simulink model "nieliniowy"  (R2013a)
settings: Solver=ode45  SolverMode=SingleTasking  StartTime=0.0  StopTime=4  RelTol=1e-3
values from neighbouring files (symbols this model uses):
  a = a-b    (= 0.0214)    [model_nielin_zmienne.m]    (also in model_nieliniowy_zmienne.m = 0.0928)
  b = a-b    (= 0.0928)    [model_nielin_zmienne.m]    (also in model_nieliniowy_zmienne.m = 0.0214)
  g = 9.81    [model_nielin_zmienne.m]    (also in model_nieliniowy_zmienne.m)
  k = 0.2607    [model_nielin_zmienne.m]    (also in model_nieliniowy_zmienne.m)
  m = 58    [model_nielin_zmienne.m]    (also in model_nieliniowy_zmienne.m)
  T = 0.024    [model_nielin_zmienne.m]    (also in model_nieliniowy_zmienne.m)
  u_c = -0.0062    [model_nielin_zmienne.m]    (also in model_nieliniowy_zmienne.m)
  x10 = 0.010    (= 0.01)    [model_nielin_zmienne.m]    (also in model_nieliniowy_zmienne.m = 0.013)
  x1zad = 0.012    [model_nielin_zmienne.m]    (also in model_nieliniowy_zmienne.m = 0.014)
  x20 = -1e-10    [model_nielin_zmienne.m]    (also in model_nieliniowy_zmienne.m = -1e-09)
  x30 = 1e-9    (= 1e-09)    [model_nielin_zmienne.m]    (also in model_nieliniowy_zmienne.m)
undefined symbols (not defined in the file or in its folder): K
libraries: simulink x2
settings Model: Creator=piotr  LastModifiedBy=Filip
settings DataIOCC: SignalLoggingSaveFormat=ModelDataLogs
settings OptimizationCC: BlockReduction=off  BooleanDataType=off
settings DebuggingCC: SaveWithParameterizedLinksMsg=none  SignalResolutionControl=TryResolveAllWithWarning  SolverPrmCheckMsg=none  MultiTaskDSMMsg=warning  MultiTaskCondExecSysMsg=none  StrictBusMsg=None
settings HardwareCC: TargetUnknown=on
settings RTWCC: IncludeERTFirstTime=on

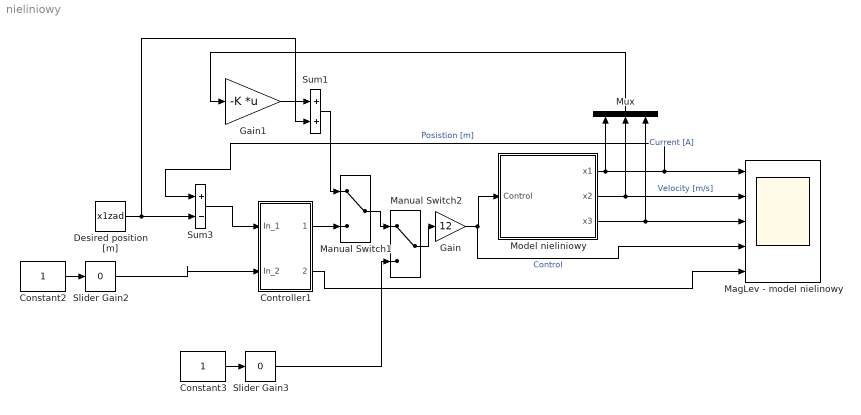
== system nieliniowy ==
  Constant2 : Constant
  Constant3 : Constant
  Controller1 : Subsystem  mask(PID(2) Controller){P=40, I=3, D=0.5, T0=0.001}
      mask prompts: P "Proportional:"; I "Integral:"; D "Derivative:"; T0 "Sample Time:"
      mask help:
      | Enter Proportional(P), Integral(I), and Derivative(D) and divisor (N) terms.
      | P+I/s+Ds/(1/Ns+1)
      mask Help: This block implements a PID controller where parameters are entered for the Proportional, Integral and Derivative and divisor terms. Unmask this block to see how it works. The derivative term is implemented using an s/(s/N +1)  transfer function block. Making N large can create a "stiff" system.
      mask Display: disp('PID')
  "Desired position [m] " : Constant  Value=x1zad
  Gain : Gain  Gain=12
  Gain1 : Gain  Gain=-K  Multiplication=Matrix(K*u)
  MagLev - model nielinowy : Scope  NumInputPorts=5
      settings: TimeRange=100  YMin=-0.45~-0.1~-0.1~0~-5  YMax=0.15~0.125~1.5~6.5~5  SaveName=ModelNieliniowy  MaxDataPoints=10000
  Manual Switch1 : ManualSwitch
  Manual Switch2 : ManualSwitch
  Model nieliniowy : Subsystem
  Mux : Mux  Inputs=3
  Slider Gain2 : simulink/Math Operations/Slider Gain  low=0  gain=0  high=1
  Slider Gain3 : simulink/Math Operations/Slider Gain  low=0  gain=0  high=1
  Sum1 : Sum  SaturateOnIntegerOverflow=on  InputSameDT=on  OutDataTypeStr=Inherit: Same as first input
  Sum3 : Sum  Inputs=+-  SaturateOnIntegerOverflow=on  InputSameDT=on  OutDataTypeStr=Inherit: Same as first input
  wires:
  Model nieliniowy/1(x1) -> Sum3/1, MagLev - model nielinowy/1, Mux/1  "Posistion [m]"
  Model nieliniowy/2(x2) -> MagLev - model nielinowy/2, Mux/2  "Velocity [m/s]"
  Model nieliniowy/3(x3) -> MagLev - model nielinowy/3, Mux/3  "Current [A]"
  Constant2/1 -> Slider Gain2/1
  Slider Gain2/1 -> Controller1/2(In_2)
  "Desired position [m] "/1 -> Sum1/2, Sum3/2
  Sum3/1 -> Controller1/1(In_1)
  Gain/1 -> Model nieliniowy/1(Control), MagLev - model nielinowy/4  "Control"
  Constant3/1 -> Slider Gain3/1
  Slider Gain3/1 -> Manual Switch2/2
  Manual Switch2/1 -> Gain/1
  Controller1/2(Out_2) -> MagLev - model nielinowy/5
  Manual Switch1/1 -> Manual Switch2/1
  Controller1/1(Out_1) -> Manual Switch1/2
  Mux/1 -> Gain1/1
  Gain1/1 -> Sum1/1
  Sum1/1 -> Manual Switch1/1

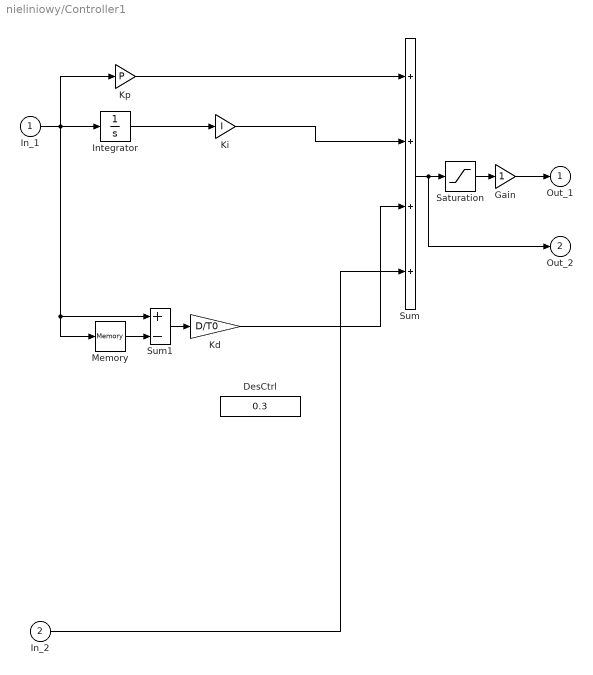
== system nieliniowy/Controller1 ==
  In_1 : Inport
  In_2 : Inport  Port=2
  DesCtrl : Constant  Value=0.3
  Gain : Gain  SaturateOnIntegerOverflow=on  OutDataTypeStr=Inherit: Same as input  ParamDataTypeStr=Inherit: Same as input
  Integrator : Integrator  InitialCondition=0*4e-5  LimitOutput=on  UpperSaturationLimit=1  LowerSaturationLimit=-1
  Kd : Gain  Gain=D/T0  SaturateOnIntegerOverflow=on  OutDataTypeStr=Inherit: Same as input  ParamDataTypeStr=Inherit: Same as input
  Ki : Gain  Gain=I  SaturateOnIntegerOverflow=on  OutDataTypeStr=Inherit: Same as input  ParamDataTypeStr=Inherit: Same as input
  Kp : Gain  Gain=P  SaturateOnIntegerOverflow=on  OutDataTypeStr=Inherit: Same as input  ParamDataTypeStr=Inherit: Same as input
  Memory : Memory
  Saturation : Saturate  UpperLimit=1  LowerLimit=0
  Sum : Sum  Inputs=++++  SaturateOnIntegerOverflow=on  InputSameDT=on  OutDataTypeStr=Inherit: Same as first input
  Sum1 : Sum  Inputs=+-  SaturateOnIntegerOverflow=on  InputSameDT=on  OutDataTypeStr=Inherit: Same as first input
  Out_1 : Outport  InitialOutput=0
  Out_2 : Outport  Port=2  InitialOutput=0
  wires:
  In_2/1 -> Sum/4
  Gain/1 -> Out_1/1
  Kd/1 -> Sum/3
  Kp/1 -> Sum/1
  Saturation/1 -> Gain/1
  Sum1/1 -> Kd/1
  Memory/1 -> Sum1/2
  In_1/1 -> Integrator/1, Sum1/1, Memory/1, Kp/1
  Sum/1 -> Out_2/1, Saturation/1
  Integrator/1 -> Ki/1
  Ki/1 -> Sum/2

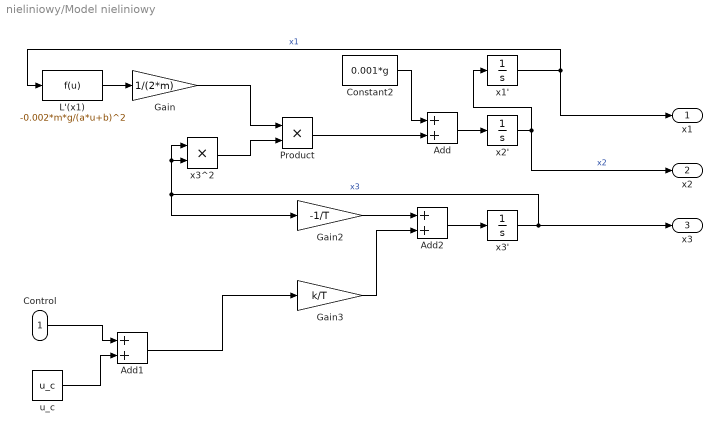
== system nieliniowy/Model nieliniowy ==
  Control : Inport
  Add : Sum
  Add1 : Sum
  Add2 : Sum
  Constant2 : Constant  Value=0.001*g
  Gain : Gain  Gain=1/(2*m)
  Gain2 : Gain  Gain=-1/T
  Gain3 : Gain  Gain=k/T
  L'(x1) : Fcn  Expr=-0.002*m*g/(a*u+b)^2
  Product : Product
  u_c : Constant  Value=u_c
  x1' : Integrator  InitialCondition=x10  LimitOutput=on  UpperSaturationLimit=0.03  LowerSaturationLimit=0
  x2' : Integrator  InitialCondition=x20
  x3' : Integrator  InitialCondition=x30  LimitOutput=on  UpperSaturationLimit=10  LowerSaturationLimit=0
  x3^2 : Product
  x1 : Outport
  x2 : Outport  Port=2
  x3 : Outport  Port=3
  wires:
  Control/1 -> Add1/1
  x1'/1 -> x1/1, L'(x1)/1  "x1"
  L'(x1)/1 -> Gain/1
  x3'/1 -> Gain2/1, x3^2/2, x3^2/1, x3/1  "x3"
  Gain/1 -> Product/1
  x3^2/1 -> Product/2
  x2'/1 -> x2/1, x1'/1  "x2"
  Add/1 -> x2'/1
  Constant2/1 -> Add/1
  Product/1 -> Add/2
  Add2/1 -> x3'/1
  u_c/1 -> Add1/2
  Add1/1 -> Gain3/1
  Gain2/1 -> Add2/1
  Gain3/1 -> Add2/2
